simulink model "MOSFET_model"  (R2016a)
settings: Solver=VariableStepAuto  StartTime=0.0  StopTime=10.0  RelTol=1e-3
libraries: elec_lib x5, fl_lib x4, nesl_utility x1
settings Model: Creator=syf  LastModifiedBy=syf

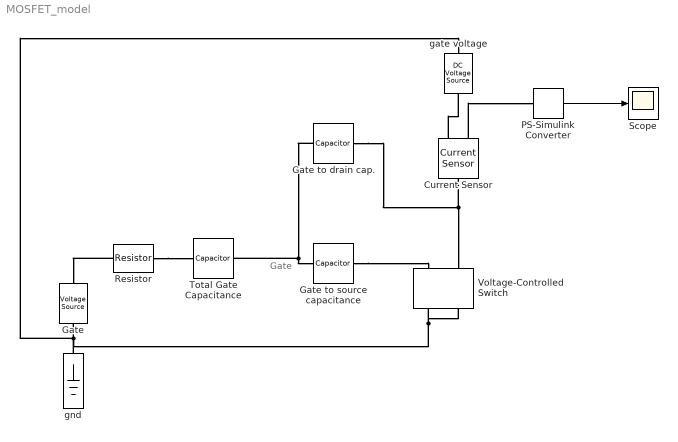
== system MOSFET_model ==
  note: Gate
  Current Sensor : fl_lib/Electrical/Electrical Sensors/Current Sensor
  Gate : elec_lib/Sources/Voltage Source  dc_voltage=0 V  ac_voltage=5 V  ac_shift=0 deg  ac_frequency=60 Hz  noise_mode=0  PSD=0 V^2/Hz  sample_time=0.001 s  repeatability=1  auto_seed=993158858  user_seed=0
  Gate to drain cap. : elec_lib/Passive Devices/Capacitor  enable_table=0  c=0.3 nF  Cvec=[ 1e-5 1e-6 ] F  Vvec=[ 0 10 ] V  CV_table_symmetry=1  C_tol=5  enable_C_tol=0  tol_distribution=1  nSigma=4  r=1e-6 Ohm  g=0 1/Ohm  initV=0 V  enable_operating_limits=0  operating_limit_action=2  max_working_voltage_range=[ -25 25 ] V  power_rating=1 W  enable_faults=0  fault_action=1  Cscale_faulted=100  R_faulted=0.001 Ohm  G_faulted=0 1/Ohm  tau_fault=0.001 s  enable_temporal_fault=0  t_fault=1 s  enable_behavioral_fault=0  max_permissible_voltage_range=[ -100 100 ] V  t_fail_on_voltage=1 s
  Gate to source capacitance : elec_lib/Passive Devices/Capacitor  enable_table=0  c=2.2/6 nF  Cvec=[ 1e-5 1e-6 ] F  Vvec=[ 0 10 ] V  CV_table_symmetry=1  C_tol=5  enable_C_tol=0  tol_distribution=1  nSigma=4  r=1e-6 Ohm  g=0 1/Ohm  initV=0 V  enable_operating_limits=0  operating_limit_action=2  max_working_voltage_range=[ -25 25 ] V  power_rating=1 W  enable_faults=0  fault_action=1  Cscale_faulted=100  R_faulted=0.001 Ohm  G_faulted=0 1/Ohm  tau_fault=0.001 s  enable_temporal_fault=0  t_fault=1 s  enable_behavioral_fault=0  max_permissible_voltage_range=[ -100 100 ] V  t_fail_on_voltage=1 s
  PS-Simulink Converter : nesl_utility/PS-Simulink Converter  PhysicalDomain=network_engine_domain  SubClassName=ps_output  LeftPortType=input  RightPortType=output  PseudoPeriodic=off  Frequencies=[]  Unit=1  AffineConversion=off
  Resistor : fl_lib/Electrical/Electrical Elements/Resistor  R=1.5 Ohm  i_specify=off  i_priority=None  i=0 A  v_specify=off  v_priority=None  v=0 V
  Scope : Scope
  Total Gate Capacitance : elec_lib/Passive Devices/Capacitor  enable_table=0  c=5.8/6 nF  Cvec=[ 1e-5 1e-6 ] F  Vvec=[ 0 10 ] V  CV_table_symmetry=1  C_tol=5  enable_C_tol=0  tol_distribution=1  nSigma=4  r=1e-6 Ohm  g=0 1/Ohm  initV=0 V  enable_operating_limits=0  operating_limit_action=2  max_working_voltage_range=[ -25 25 ] V  power_rating=1 W  enable_faults=0  fault_action=1  Cscale_faulted=100  R_faulted=0.001 Ohm  G_faulted=0 1/Ohm  tau_fault=0.001 s  enable_temporal_fault=0  t_fault=1 s  enable_behavioral_fault=0  max_permissible_voltage_range=[ -100 100 ] V  t_fail_on_voltage=1 s
  Voltage-Controlled Switch : elec_lib/Additional Components/SPICE-Compatible Components/Passive Devices/Voltage-Controlled Switch  VT=1.3 V  VH=0 V  RON=160 Ohm  ROFF=1e+12 Ohm  IC_state=-1
  gate voltage : fl_lib/Electrical/Electrical Sources/DC Voltage Source  v0=5 V
  gnd : fl_lib/Electrical/Electrical Elements/Electrical Reference
  wires:
  PS-Simulink Converter/1 -> Scope/1
  connections:
  gnd/LConn1 -- gate voltage/RConn1 -- Gate/RConn1 -- Voltage-Controlled Switch/RConn2 -- Voltage-Controlled Switch/RConn1
  Gate to drain cap./LConn1 -- Gate to source capacitance/LConn1 -- Total Gate Capacitance/RConn1
  Resistor/RConn1 -- Total Gate Capacitance/LConn1
  Resistor/LConn1 -- Gate/LConn1
  Gate to source capacitance/RConn1 -- Voltage-Controlled Switch/LConn1
  Gate to drain cap./RConn1 -- Current Sensor/LConn1 -- Voltage-Controlled Switch/LConn2
  Current Sensor/RConn2 -- gate voltage/LConn1
  Current Sensor/RConn1 -- PS-Simulink Converter/LConn1
